simulink model "PV_PEM_direct_battery_passive"  (R2026a)
settings: Solver=VariableStepAuto  StopTime=sim_t
values from neighbouring files (symbols this model uses):
  Irr_stair_time = (0:Irr_stair_tsamp:sim_t)'    [PV_PEM_direct_battery_active.m]    (also in PV_PEM_direct_battery_passive.m = 0:Irr_stair_tsamp:sim_t; PV_PEM_indirect_battery.m; PV_PEM_reconfigurable_battery.m = (0 : Irr_stair_tsamp : sim_t)')
  Irr_stair_val = interp1(Irr_time, Irr_val, Irr_stair_time, 'linear', 0)    [PV_PEM_direct_battery_active.m]    (also in PV_PEM_direct_battery_passive.m; PV_PEM_indirect_battery.m; PV_PEM_reconfigurable_battery.m = interp1(Irr_time, Irr_val,  Irr_stair_time, 'linear', 0))
  Q_batt = 0.1    [PV_PEM_direct_battery_active.m]    (also in PV_PEM_direct_battery_passive.m; PV_PEM_indirect_battery.m; PV_PEM_reconfigurable_battery.m = 0.00694444444444)
  Ra_stack = Ra   * N    (= 0.02301)    [PV_PEM_direct_battery_active.m]    (also in PV_PEM_direct_battery_passive.m; PV_PEM_indirect_battery.m = 0.0177; PV_PEM_reconfigurable_battery.m = 0.02832)
  Rc_stack = Rc   * N    (= 0.0065)    [PV_PEM_direct_battery_active.m]    (also in PV_PEM_direct_battery_passive.m; PV_PEM_indirect_battery.m = 0.005; PV_PEM_reconfigurable_battery.m = 0.008)
  Rint_stack = Rint * N    (= 0.112749)    [PV_PEM_direct_battery_active.m]    (also in PV_PEM_direct_battery_passive.m; PV_PEM_indirect_battery.m = 0.08673; PV_PEM_reconfigurable_battery.m = 0.138768)
  sample_output_time = 1e-3    (= 0.001)    [PV_PEM_direct_battery_active.m]    (also in PV_PEM_direct_battery_passive.m = 0.0001; PV_PEM_indirect_battery.m = 0.01; PV_PEM_reconfigurable_battery.m = 0.00166666666667)
  SOC_max = 0.9    [PV_PEM_direct_battery_active.m]    (also in PV_PEM_direct_battery_passive.m = 90; PV_PEM_indirect_battery.m; PV_PEM_reconfigurable_battery.m = 90)
  SOC_min = 0.2    [PV_PEM_direct_battery_active.m]    (also in PV_PEM_direct_battery_passive.m = 20; PV_PEM_indirect_battery.m; PV_PEM_reconfigurable_battery.m = 20)
libraries: fl_lib x20, nesl_utility x15, simulink x3, ee_lib x3, batteryecm_lib x1
settings Model: Creator=hanna  LastModifiedBy=Diamantis
settings SimscapeCC: SimscapeNominalValues="[{\"value\":\"1\",\"unit\":\"A\"},{\"value\":\"1\",\"unit\":\"bar\"},{\"value\":\"1\",\"unit\":\"cm^2\"},{\"value\":\"1\",\"unit\":\"cm^3/s\"},{\"value\":\"1\",\"unit\":\"kJ/kg\"},{\"value\":\"1\",\"unit\":\"kW\"},{\"value\":\"1\",\"unit\":\"l\"},{\"value\":\"1\",\"unit\":\"N\"},{\"value\":\"1\",\"unit\":\"N*m\"},{\"value\":\"1\",\"unit\":\"V\"}]"  SimscapeLogType=none  SimscapeLogDataHistory=5000.0

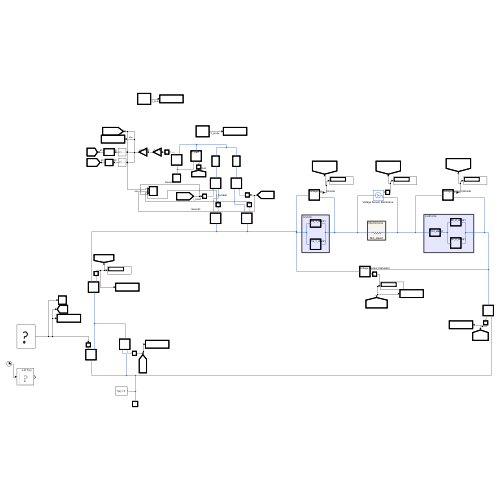
[thumbnail: Simulink's stored preview of the top-level diagram]
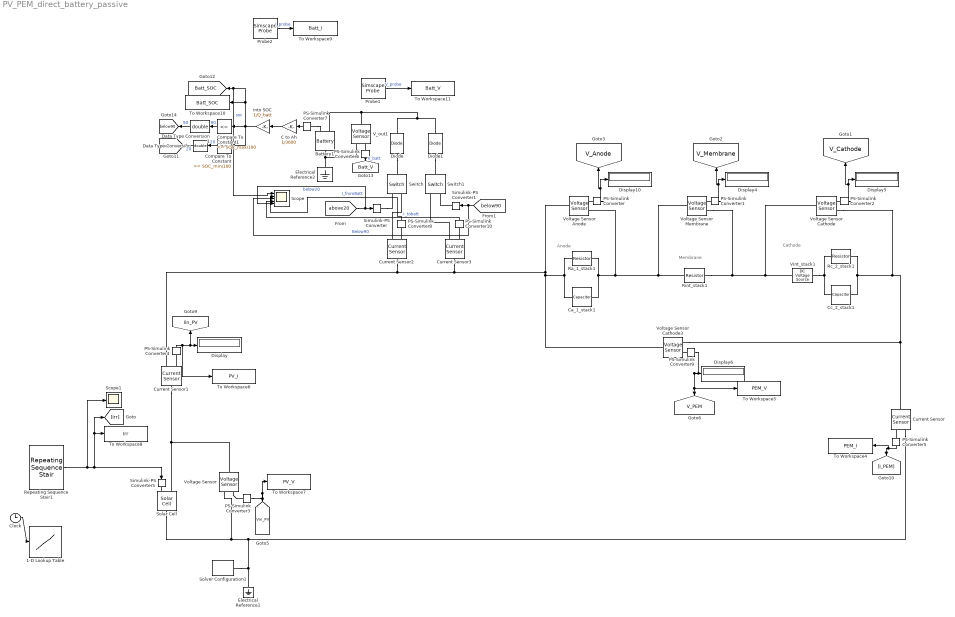
== system PV_PEM_direct_battery_passive ==
  note: Membrane
  note: Cathode
  note: Anode
  1-D Lookup Table : Lookup_n-D  NumberOfTableDimensions=1  BreakpointsForDimension1=Irr_stair_time  Table=Irr_stair_val  InternalRulePriority=Speed  RndMeth=Simplest
  Battery1 : batteryecm_lib/Battery  Vnom=V_batt_nom V  prm_dir=simscape.enum.battery.prm_dir.disabled  R1_dis=0.05 Ohm  R1_ch=0.05 Ohm  R1=0.01 Ohm  prm_AH=simscape.enum.battery.prm_AH.finite  AH=Q_batt A*hr  V1=11.5 V  AH1=Q_batt*(SOC_min/100) A*hr  prm_R2=simscape.enum.battery.prm_R2.disabled  R2=2000 Ohm  Tmeas=298.15 K  charge_measurement_port=simscape.enum.battery.enable.yes  prm_dyn=simscape.enum.battery.prm_dyn.off  Rp1=0.005 Ohm  tau1=30 s  Rp2=0.005 Ohm  tau2=30 s  Rp3=0.005 Ohm  tau3=30 s  Rp4=0.005 Ohm  tau4=30 s  Rp5=0.005 Ohm  tau5=30 s  prm_fade=simscape.enum.battery.prm_fade.disabled  N_fade=100  AH_fade=45 A*hr  R1_fade=2.02 Ohm  R1_ch_fade=2.02 Ohm  V1_fade=10.35 V  prm_age=simscape.enum.battery.prm_age.disabled  prm_age_OCV=simscape.enum.battery.prm_age_OCV.OCV  OCV_age=0.9  SOC_age=60  Tmeas_age=298.15 K  delta_time_age_vec=[0] d  temperature_age_vec=[273] K  OCV_scaling_age=2.2134e6  OCV_offset_age=1.632e6  temp_exp_age=0.515833569 V  t_exp_age=0.75  Vnom_T2=12 V  R1_T2=2.2 Ohm  R1_T2_dis=2.2 Ohm  R1_T2_ch=2.2 Ohm  V1_T2=11.4 V  R2_T2=2200 Ohm  Rp1_T2=0.005 Ohm  tau1_T2=30 s  Rp2_T2=0.005 Ohm  tau2_T2=30 s  Rp3_T2=0.005 Ohm  tau3_T2=30 s  Rp4_T2=0.005 Ohm  tau4_T2=30 s  Rp5_T2=0.005 Ohm  tau5_T2=30 s  Tmeas2=273.15 K  thermal_port=simscape.enum.thermaleffects.omit  thermal_mass=30000 J/K  i_specify=off  i_priority=None  i=0 A  i_nominal_specify=off  i_nominal_value=1  i_nominal_unit=A  v_specify=off  v_priority=None  v=0 V  v_nominal_specify=off  v_nominal_value=1  v_nominal_unit=V  charge_specify=on  charge_priority=High  charge=SOC_init A*hr  charge_nominal_specify=off  charge_nominal_value=1  charge_nominal_unit=A*hr  num_cycles_specify=off  num_cycles_priority=High  num_cycles=0  num_cycles_nominal_specify=off  num_cycles_nominal_value=1  num_cycles_nominal_unit=1  temperature_specify=off  temperature_priority=High  temperature=298.15 K  temperature_nominal_specify=off  temperature_nominal_value=1  temperature_nominal_unit=K
      settings: LibrarySourceBlock=batt_lib/Cells/Battery
  C to Ah : Gain  Gain=1/3600
  Ca_1_stack1 : fl_lib/Electrical/Electrical Elements/Capacitor  c=Ca_stack F  r=1e-6 Ohm  g=0 1/Ohm  i_specify=off  i_priority=None  i=0 A  i_nominal_specify=off  i_nominal_value=1  i_nominal_unit=A  v_specify=off  v_priority=None  v=0 V  v_nominal_specify=off  v_nominal_value=1  v_nominal_unit=V  vc_specify=off  vc_priority=High  vc=0 V  vc_nominal_specify=off  vc_nominal_value=1  vc_nominal_unit=V
  Cc_2_stack1 : fl_lib/Electrical/Electrical Elements/Capacitor  c=Cc_stack F  r=1e-6 Ohm  g=0 1/Ohm  i_specify=off  i_priority=None  i=0 A  i_nominal_specify=off  i_nominal_value=1  i_nominal_unit=A  v_specify=off  v_priority=None  v=0 V  v_nominal_specify=off  v_nominal_value=1  v_nominal_unit=V  vc_specify=off  vc_priority=High  vc=0 V  vc_nominal_specify=off  vc_nominal_value=1  vc_nominal_unit=V
  Clock : Clock
  Compare To Constant : simulink/Logic and Bit Operations/Compare To Constant  relop=>=  const=SOC_min/100  OutDataTypeStr=boolean
  Compare To Constant1 : simulink/Logic and Bit Operations/Compare To Constant  relop=<=  const=SOC_max/100  OutDataTypeStr=boolean
  Current Sensor{,1..3} (4 alike) : fl_lib/Electrical/Electrical Sensors/Current Sensor
  Data Type Conversion : DataTypeConversion  OutDataTypeStr=double  SaturateOnIntegerOverflow=off  RndMeth=Floor
  Data Type Conversion1 : DataTypeConversion  OutDataTypeStr=double  SaturateOnIntegerOverflow=off  RndMeth=Floor
  Diode : ee_lib/Semiconductors & Converters/Diode  ModelType=ee.enum.diode.modelType.pwl  TableType=ee.enum.diode.tableType.IfMat  IfMat=[.07, .12, .19, 1.75, 4.24, 7.32, 11.2; .16, .3, .72, 2.14, 5.02, 8.35, 13.12] A  VfMat=[.9, 1.15, 1.25, 1.5, 1.75, 2.17, 2.6, 2.85; .58, .68, .75, 1.1, 1.38, 1.77, 2.27, 2.7] V  TjVec=[25, 125] degC  VfVec=[.5, .7, .9, 1.3, 1.7, 2.1, 2.5] V  IfVec=[.1, .2, .5, 1, 2, 4, 7, 10] A  IrMat=[1e-06, 2e-06, 5e-06, 1e-05, 2.5e-05, 5e-05, .0001; 2e-06, 5e-06, 1e-05, 4e-05, 8e-05, .0002, .0005] A  VrMat=[10, 100, 200, 250, 300, 325, 350; 10, 70, 160, 220, 270, 300, 320] V  VrVec=[10, 20, 40, 50, 70, 80, 100] V  IrVec=[1e-06, 2e-06, 5e-06, 1e-05, 2e-05, 5e-05, .0001] A  Vf=0.6 V  Ron=0.3 Ohm  Goff=1e-8 S  prmExp=ee.enum.diode.expParam.useTwo  I12=[.0137, .545] A  V12=[.6, .7] V  RS=0 Ohm  Tmeas=298.15 K  IS=1e-12 A  ec=1  I1=0.0137 A  V1=0.6 V  N_series=1  N_parallel=1  ZenerEnable=false  Rz=0.3 Ohm  BV=inf V  C_param=ee.enum.diode.capParam.fixed  CJ=0 pF  CJ0=5 pF  Vvec=[.1, 10, 100] V  Cvec=[3.5, 1, .4] pF  VJ=1 V  Mgrad=0.5  FC=0.5  Q_param=ee.enum.diode.recoveryParam.off  iRM=-7.15 A  iF=4 A  didt=-750 A/us  trr_factor=3  trr=115 ns  Qrr=150 nA*s  Vr=-600 V  Ls=150 nH  Erec=0.03 J  TT=50 ns  tau=100 ns  T_param=ee.enum.diode.temperatureParam.off  Tdevice=298.15 K  I1_T2=0.245 A  V1_T2=0.5 V  IS_T2=1.25e-7 A  Tmeas2=125 degC  XTI_param=ee.enum.diode.xtiParam.pn  XTI=3  EG_param=ee.enum.diode.egapParam.material_si  EG=1.11 eV  dBVdT=0 V/K  enable_fault_input=simscape.enum.onoff.off  i_specify=off  i_priority=None  i=0 A  i_nominal_specify=off  i_nominal_value=1  i_nominal_unit=A  v_specify=off  v_priority=None  v=0 V  v_nominal_specify=off  v_nominal_value=1  v_nominal_unit=V  v_capacitor_specify=off  v_capacitor_priority=None  v_capacitor=0 V  v_capacitor_nominal_specify=off  v_capacitor_nominal_value=1  v_capacitor_nominal_unit=V  Qj_specify=off  Qj_priority=High  Qj=0 C  Qj_nominal_specify=off  Qj_nominal_value=1  Qj_nominal_unit=C  i_diode_specify=off  i_diode_priority=None  i_diode=0 A  i_diode_nominal_specify=off  i_diode_nominal_value=1  i_diode_nominal_unit=A  v_diode_specify=off  v_diode_priority=None  v_diode=0 V  v_diode_nominal_specify=off  v_diode_nominal_value=1  v_diode_nominal_unit=V  i_capacitor_specify=off  i_capacitor_priority=None  i_capacitor=0 A  i_capacitor_nominal_specify=off  i_capacitor_nominal_value=1  i_capacitor_nominal_unit=A  fidelity_level=ee.enum.diode.fidelity.includeChargeDyn  rec_loss_model=ee.enum.diode.reverseRecoveryModel.fixed  ErecVal=0 J  scaleWithIandV=true  ErecMat=zeros(2, 3) J  ErecMat3D=zeros(2, 3, 2) J  TjrecVec=[298.15, 398.15] K  IfrecVec=[.1, 1, 10] A  IrecVal=10 A  VrecVal=10 V  VrecVec=[0, 100] V  tFilter=1 / 1000 / 100 s  thermal_network_parameterization=ee.enum.thermalNetworkTopology.junctionCase  Rth=[0, 10] K/W  Rth_Cauer=[1, 3, 10] K/W  Rth_Foster=[.08, .14, .22, .16] K/W  thermal_mass_parameterization=ee.enum.thermalNetwork.timeconstant  thermal_mass=[0, 1] J/K  thermal_mass_Cauer=[.1, .3, 1] J/K  thermal_mass_Foster=[.001, .005, .05, .5] J/K  thermal_time_constant=[0, 10] s  thermal_time_constant_Cauer=[1, 3, 10] s  thermal_time_constant_Foster=[7e-05, .0007, .01, .08] s  thermal_mass_initial_temperatures=[25, 25] degC  thermal_mass_initial_temperatures_Cauer=[25, 25, 25] degC  junction_thermal_mass=0.01 J/K  Tvec_initial_Foster=[25, 25, 25, 25] degC  no_thermal_network=0  junction_temperature_specify=off  junction_temperature_priority=None  junction_temperature=25 degC  junction_temperature_nominal_specify=off  junction_temperature_nominal_value=1  junction_temperature_nominal_unit=degC
  Diode1 : ee_lib/Semiconductors & Converters/Diode  ModelType=ee.enum.diode.modelType.pwl  TableType=ee.enum.diode.tableType.IfMat  IfMat=[.07, .12, .19, 1.75, 4.24, 7.32, 11.2; .16, .3, .72, 2.14, 5.02, 8.35, 13.12] A  VfMat=[.9, 1.15, 1.25, 1.5, 1.75, 2.17, 2.6, 2.85; .58, .68, .75, 1.1, 1.38, 1.77, 2.27, 2.7] V  TjVec=[25, 125] degC  VfVec=[.5, .7, .9, 1.3, 1.7, 2.1, 2.5] V  IfVec=[.1, .2, .5, 1, 2, 4, 7, 10] A  IrMat=[1e-06, 2e-06, 5e-06, 1e-05, 2.5e-05, 5e-05, .0001; 2e-06, 5e-06, 1e-05, 4e-05, 8e-05, .0002, .0005] A  VrMat=[10, 100, 200, 250, 300, 325, 350; 10, 70, 160, 220, 270, 300, 320] V  VrVec=[10, 20, 40, 50, 70, 80, 100] V  IrVec=[1e-06, 2e-06, 5e-06, 1e-05, 2e-05, 5e-05, .0001] A  Vf=0.6 V  Ron=0.3 Ohm  Goff=1e-8 S  prmExp=ee.enum.diode.expParam.useTwo  I12=[.0137, .545] A  V12=[.6, .7] V  RS=0 Ohm  Tmeas=298.15 K  IS=1e-12 A  ec=1  I1=0.0137 A  V1=0.6 V  N_series=1  N_parallel=1  ZenerEnable=false  Rz=0.3 Ohm  BV=inf V  C_param=ee.enum.diode.capParam.fixed  CJ=0 pF  CJ0=5 pF  Vvec=[.1, 10, 100] V  Cvec=[3.5, 1, .4] pF  VJ=1 V  Mgrad=0.5  FC=0.5  Q_param=ee.enum.diode.recoveryParam.off  iRM=-7.15 A  iF=4 A  didt=-750 A/us  trr_factor=3  trr=115 ns  Qrr=150 nA*s  Vr=-600 V  Ls=150 nH  Erec=0.03 J  TT=50 ns  tau=100 ns  T_param=ee.enum.diode.temperatureParam.off  Tdevice=298.15 K  I1_T2=0.245 A  V1_T2=0.5 V  IS_T2=1.25e-7 A  Tmeas2=125 degC  XTI_param=ee.enum.diode.xtiParam.pn  XTI=3  EG_param=ee.enum.diode.egapParam.material_si  EG=1.11 eV  dBVdT=0 V/K  enable_fault_input=simscape.enum.onoff.off  i_specify=off  i_priority=None  i=0 A  i_nominal_specify=off  i_nominal_value=1  i_nominal_unit=A  v_specify=off  v_priority=None  v=0 V  v_nominal_specify=off  v_nominal_value=1  v_nominal_unit=V  v_capacitor_specify=off  v_capacitor_priority=None  v_capacitor=0 V  v_capacitor_nominal_specify=off  v_capacitor_nominal_value=1  v_capacitor_nominal_unit=V  Qj_specify=off  Qj_priority=High  Qj=0 C  Qj_nominal_specify=off  Qj_nominal_value=1  Qj_nominal_unit=C  i_diode_specify=off  i_diode_priority=None  i_diode=0 A  i_diode_nominal_specify=off  i_diode_nominal_value=1  i_diode_nominal_unit=A  v_diode_specify=off  v_diode_priority=None  v_diode=0 V  v_diode_nominal_specify=off  v_diode_nominal_value=1  v_diode_nominal_unit=V  i_capacitor_specify=off  i_capacitor_priority=None  i_capacitor=0 A  i_capacitor_nominal_specify=off  i_capacitor_nominal_value=1  i_capacitor_nominal_unit=A  fidelity_level=ee.enum.diode.fidelity.includeChargeDyn  rec_loss_model=ee.enum.diode.reverseRecoveryModel.fixed  ErecVal=0 J  scaleWithIandV=true  ErecMat=zeros(2, 3) J  ErecMat3D=zeros(2, 3, 2) J  TjrecVec=[298.15, 398.15] K  IfrecVec=[.1, 1, 10] A  IrecVal=10 A  VrecVal=10 V  VrecVec=[0, 100] V  tFilter=1 / 1000 / 100 s  thermal_network_parameterization=ee.enum.thermalNetworkTopology.junctionCase  Rth=[0, 10] K/W  Rth_Cauer=[1, 3, 10] K/W  Rth_Foster=[.08, .14, .22, .16] K/W  thermal_mass_parameterization=ee.enum.thermalNetwork.timeconstant  thermal_mass=[0, 1] J/K  thermal_mass_Cauer=[.1, .3, 1] J/K  thermal_mass_Foster=[.001, .005, .05, .5] J/K  thermal_time_constant=[0, 10] s  thermal_time_constant_Cauer=[1, 3, 10] s  thermal_time_constant_Foster=[7e-05, .0007, .01, .08] s  thermal_mass_initial_temperatures=[25, 25] degC  thermal_mass_initial_temperatures_Cauer=[25, 25, 25] degC  junction_thermal_mass=0.01 J/K  Tvec_initial_Foster=[25, 25, 25, 25] degC  no_thermal_network=0  junction_temperature_specify=off  junction_temperature_priority=None  junction_temperature=25 degC  junction_temperature_nominal_specify=off  junction_temperature_nominal_value=1  junction_temperature_nominal_unit=degC
  Display{,4..6,10} (5 alike) : Display
  Electrical Reference2 : fl_lib/Electrical/Electrical Elements/Electrical Reference
  Electrical Reference1 : fl_lib/Electrical/Electrical Elements/Electrical Reference
  PS-Simulink Converter{,1..2,5..7,9} (7 alike) : nesl_utility/PS-Simulink Converter  PhysicalDomain=network_engine_domain  SubClassName=ps_output  LeftPortType=input  RightPortType=output  PseudoPeriodic=off  Frequencies=[]  VectorFormat=inherit  Unit=inherit  AffineConversion=off
  PS-Simulink Converter10 : nesl_utility/PS-Simulink Converter  PhysicalDomain=network_engine_domain  SubClassName=ps_output  LeftPortType=input  RightPortType=output  PseudoPeriodic=off  Frequencies=[]  VectorFormat=1-D array  Unit=A  AffineConversion=off
  PS-Simulink Converter3 : nesl_utility/PS-Simulink Converter  PhysicalDomain=network_engine_domain  SubClassName=ps_output  LeftPortType=input  RightPortType=output  PseudoPeriodic=off  Frequencies=[]  VectorFormat=1-D array  Unit=V  AffineConversion=off
  PS-Simulink Converter4 : nesl_utility/PS-Simulink Converter  PhysicalDomain=network_engine_domain  SubClassName=ps_output  LeftPortType=input  RightPortType=output  PseudoPeriodic=off  Frequencies=[]  VectorFormat=1-D array  Unit=A  AffineConversion=off
  PS-Simulink Converter8 : nesl_utility/PS-Simulink Converter  PhysicalDomain=network_engine_domain  SubClassName=ps_output  LeftPortType=input  RightPortType=output  PseudoPeriodic=off  Frequencies=[]  VectorFormat=1-D array  Unit=A  AffineConversion=off
  Probe1 : SimscapeProbe  BoundBlock=499  Variables="{\"i\":{\"Probing\":\"OFF\"},\"n.v\":{\"Probing\":\"OFF\"},\"p.v\":{\"Probing\":\"OFF\"},\"v\":{\"Probing\":\"ON\"}}"
  Probe2 : SimscapeProbe  BoundBlock=499  Variables="{\"i\":{\"Probing\":\"ON\"}}"
  Ra_1_stack1 : fl_lib/Electrical/Electrical Elements/Resistor  R=Ra_stack Ohm  i_specify=off  i_priority=None  i=0 A  i_nominal_specify=off  i_nominal_value=1  i_nominal_unit=A  v_specify=off  v_priority=None  v=0 V  v_nominal_specify=off  v_nominal_value=1  v_nominal_unit=V
  Rc_2_stack1 : fl_lib/Electrical/Electrical Elements/Resistor  R=Rc_stack Ohm  i_specify=off  i_priority=None  i=0 A  i_nominal_specify=off  i_nominal_value=1  i_nominal_unit=A  v_specify=off  v_priority=None  v=0 V  v_nominal_specify=off  v_nominal_value=1  v_nominal_unit=V
  Repeating Sequence Stair1 : simulink/Sources/Repeating Sequence Stair  OutValues=Irr_stair_val  tsamp=Irr_stair_tsamp  OutMin=[]  OutMax=[]  OutDataTypeStr=double  OutputDataTypeScalingMode=double  OutDataType=fixdt(0,8)  ConRadixGroup=Best Precision: Vector-wise  OutScaling=2^-12
  Rint_stack1 : fl_lib/Electrical/Electrical Elements/Resistor  R=Rint_stack Ohm  i_specify=off  i_priority=None  i=0 A  i_nominal_specify=off  i_nominal_value=1  i_nominal_unit=A  v_specify=off  v_priority=None  v=0 V  v_nominal_specify=off  v_nominal_value=1  v_nominal_unit=V
  Scope : Scope  NumInputPorts=5
      settings: ActiveDisplayYMinimum=0.599999044089406  ActiveDisplayYMaximum=0.60000010621228816  DataLoggingVariableName=ScopeData4
  Scope1 : Scope
      settings: ActiveDisplayYMinimum=-124.99999999999997  ActiveDisplayYMaximum=1125
  Simulink-PS Converter : nesl_utility/Simulink-PS Converter  PhysicalDomain=network_engine_domain  SubClassName=ps_input  LeftPortType=input  RightPortType=output  PseudoPeriodic=off  Frequencies=[]  NoiseDistribution=none  NoiseParameters=[]  Unit=1  AffineConversion=off  FilteringAndDerivatives=provide  SimscapeFilterOrder=1  InputFilterTimeConstant=0.001  UdotUserProvided=0
  Simulink-PS Converter1 : nesl_utility/Simulink-PS Converter  PhysicalDomain=network_engine_domain  SubClassName=ps_input  LeftPortType=input  RightPortType=output  PseudoPeriodic=off  Frequencies=[]  NoiseDistribution=none  NoiseParameters=[]  Unit=1  AffineConversion=off  FilteringAndDerivatives=provide  SimscapeFilterOrder=1  InputFilterTimeConstant=0.001  UdotUserProvided=0
  Simulink-PS Converter5 : nesl_utility/Simulink-PS Converter  PhysicalDomain=network_engine_domain  SubClassName=ps_input  LeftPortType=input  RightPortType=output  PseudoPeriodic=off  Frequencies=[]  NoiseDistribution=none  NoiseParameters=[]  Unit=1  AffineConversion=off  FilteringAndDerivatives=provide  SimscapeFilterOrder=1  InputFilterTimeConstant=0.001  UdotUserProvided=0
  Solar Cell : ee_lib/Sources/Solar Cell  PartSpecification="{\"CollectionId\":\"SimscapeElectrical\",\"CollectionVersion\":\"1.0.0\",\"DatasetId\":\"Amerisolar|AS_6M30_HC_320W|simscape.electrical.solarCell\",\"DisplayName\":\"Amerisolar:AS_6M30_HC_320W\"}"  prm=3  Isc=10.14 % Datasheet derived A  Voc=0.67 % Datasheet derived V  Is=3.24823447983853e-07 % Datasheet derived A  Is2=9.37081970792037e-10 % Datasheet derived A  Iph=10.140005507508 % Datasheet derived A  Ir0=1000 % Datasheet derived W/m^2  ec=1.51118472243322 % Datasheet derived  N2=2.60259908345858 % Datasheet derived  Rs=1.94548269975201e-05 % Datasheet derived Ohm  Rp=682.95993142779 % Datasheet derived Ohm  N_series=Ns_cell % Datasheet derived  N_parallel=Np_cell % Datasheet derived  TIPH1=0.000499942933005141 % Datasheet derived 1/K  EG=1.12 % Datasheet derived eV  TXIS1=4.23641510120988 % Datasheet derived  TXIS2=16.2689137700667 % Datasheet derived  TRS1=0.243341028305912 % Datasheet derived  TRP1=0 % Parameter not set  Tmeas=25 % Datasheet derived degC  TFIXED=25 % Datasheet derived degC  thermal_mass=100 % Parameter not set J/K  initial_temperature=25 degC
      settings: AttributesFormatString=Amerisolar:AS_6M30_HC_320W
  Solver Configuration1 : nesl_utility/Solver Configuration  PhysicalDomain=network_engine_domain  SubClassName=solver  LeftPortType=input  RightPortType=generic  Tones=[]  Harmonics=[]  SimulateNoise=off  Profile=off  UseLocalSampling=off  EnableSwitchedLinearOptims=on  FrequencyDomain=off  UseCCode=off  RelTol=0.001  AbsTol=0.001  MinStep=1e-09  ToWorkspace=off  RevertToSquareIcSolve=off  NumHomotopyIterations=100  PhasorMode=off  PhasorModeNumHarmonics=1  ConsistencySolver=NEWTON_XTOL_AFTER_FTOL  CanonicalOrdering=UNORDERED  OptimizeIntermediates=UNOPTIMIZED  IndexReductionMethod=DerivativeReplacement  DoDC=off  ResidualTolerance=1e-09  ConsistencyTolSource=GLOBAL  ConsistencyAbsTol=0.001  ConsistencyRelTol=0.001  ConsistencyTolFactor=0.001  UseLocalSolver=off  LocalSolverChoice=NE_BACKWARD_EULER_ADVANCER  ResolveIndetEquations=on  FunctionEvalNumThread=1  LocalSolverSampleTime=0.001  DoFixedCost=off  MaxNonlinIter=3  MaxModeIter=2  ComputeImpulses=off  ImpulseIterations=2  LinearAlgebra=auto  LinearAlgebraNumThread=0  EquationFormulation=NE_TIME_EF  DelaysMemoryBudget=1024  AutomaticFiltering=on  FilteringTimeConstant=0.001  PartitionStorageMethod=AS_NEEDED  PartitionMemoryBudget=1024  PartitionMethod=ROBUST  MultibodyUseLocalSolver=off  MultibodyLocalSolverChoice=ODE1  MultibodyLocalSolverSampleTime=0.001
  Switch : fl_lib/Electrical/Electrical Elements/Switch  R_closed=0.01 Ohm  G_open=1e-8 1/Ohm  Threshold=0.5  i_specify=off  i_priority=None  i=0 A  i_nominal_specify=off  i_nominal_value=1  i_nominal_unit=A  v_specify=off  v_priority=None  v=0 V  v_nominal_specify=off  v_nominal_value=1  v_nominal_unit=V
  Switch1 : fl_lib/Electrical/Electrical Elements/Switch  R_closed=0.01 Ohm  G_open=1e-8 1/Ohm  Threshold=0.5  i_specify=off  i_priority=None  i=0 A  i_nominal_specify=off  i_nominal_value=1  i_nominal_unit=A  v_specify=off  v_priority=None  v=0 V  v_nominal_specify=off  v_nominal_value=1  v_nominal_unit=V
  To Workspace10 : ToWorkspace  VariableName=Batt_SOC  SaveFormat=Timeseries  SampleTime=sample_output_time
  To Workspace11 : ToWorkspace  VariableName=Batt_V  SaveFormat=Timeseries  SampleTime=sample_output_time
  To Workspace4 : ToWorkspace  VariableName=PEM_I  SaveFormat=Timeseries  SampleTime=sample_output_time
  To Workspace5 : ToWorkspace  VariableName=PEM_V  SaveFormat=Timeseries  SampleTime=sample_output_time
  To Workspace6 : ToWorkspace  VariableName=PV_I  SaveFormat=Timeseries  SampleTime=sample_output_time
  To Workspace7 : ToWorkspace  VariableName=PV_V  SaveFormat=Timeseries  SampleTime=sample_output_time
  To Workspace8 : ToWorkspace  VariableName=Irr  SaveFormat=Timeseries  SampleTime=sample_output_time
  To Workspace9 : ToWorkspace  VariableName=Batt_I  SaveFormat=Timeseries  SampleTime=sample_output_time
  V_out1 : fl_lib/Electrical/Electrical Sensors/Voltage Sensor
  Vint_stack1 : fl_lib/Electrical/Electrical Sources/DC Voltage Source  v0=Vint_stack V
  Voltage Sensor : fl_lib/Electrical/Electrical Sensors/Voltage Sensor
  Voltage Sensor Anode : fl_lib/Electrical/Electrical Sensors/Voltage Sensor
  Voltage Sensor Cathode : fl_lib/Electrical/Electrical Sensors/Voltage Sensor
  Voltage Sensor Cathode3 : fl_lib/Electrical/Electrical Sensors/Voltage Sensor
  Voltage Sensor Membrane : fl_lib/Electrical/Electrical Sensors/Voltage Sensor
  into SOC : Gain  Gain=1/Q_batt
  tag scope: Batt_SOC=global, Batt_V=global, Iin_PV=global, V_Anode=global, V_Cathode=global, V_Membrane=global, V_PEM=global, Vin_PV=global, above20=global, below90=global
  wires:
  Repeating Sequence Stair1/1 -> Simulink-PS Converter5/1, To Workspace8/1, [Irr], Scope1/1
  Clock/1 -> 1-D Lookup Table/1
  PS-Simulink Converter1/1 -> [V_Membrane], Display4/1
  PS-Simulink Converter9/1 -> To Workspace5/1, [V_PEM], Display6/1
  PS-Simulink Converter/1 -> [V_Anode], Display10/1
  PS-Simulink Converter2/1 -> [V_Cathode], Display5/1
  PS-Simulink Converter4/1 -> To Workspace6/1, [Iin_PV], Display/1
  PS-Simulink Converter5/1 -> To Workspace4/1, [I_PEM]
  PS-Simulink Converter3/1 -> To Workspace7/1, [Vin_PV]
  Compare To Constant1/1 -> Data Type Conversion1/1  "90"
  Compare To Constant/1 -> Data Type Conversion/1  "20"
  into SOC/1 -> Compare To Constant1/1, To Workspace10/1, Scope/1, [Batt_SOC], Compare To Constant/1  "soc"
  Data Type Conversion1/1 -> [below90]  "90"
  C to Ah/1 -> into SOC/1
  Probe1/1 -> To Workspace11/1  "V_probe"
  PS-Simulink Converter7/1 -> C to Ah/1
  PS-Simulink Converter6/1 -> [Batt_V]  "V_batt"
  Data Type Conversion/1 -> [above20]  "20"
  Probe2/1 -> To Workspace9/1  "I_probe"
  [above20] -> Scope/5, Simulink-PS Converter/1  "below20"
  [below90] -> Scope/3, Simulink-PS Converter1/1  "Below90"
  PS-Simulink Converter10/1 -> Scope/4  "I_tobatt"
  PS-Simulink Converter8/1 -> Scope/2  "I_fromBatt"
  connections:
  Solver Configuration1/RConn1 -- Voltage Sensor/RConn2 -- Solar Cell/RConn1 -- Current Sensor/RConn2 -- Electrical Reference1/LConn1
  Simulink-PS Converter5/RConn1 -- Solar Cell/LConn1
  Current Sensor1/LConn1 -- Voltage Sensor/LConn1 -- Solar Cell/LConn2
  Voltage Sensor Anode/RConn2 -- Ra_1_stack1/RConn1 -- Ca_1_stack1/RConn1 -- Rint_stack1/LConn1 -- Voltage Sensor Membrane/LConn1
  Voltage Sensor Membrane/RConn2 -- Voltage Sensor Cathode/LConn1 -- Vint_stack1/LConn1 -- Rint_stack1/RConn1
  Cc_2_stack1/RConn1 -- Rc_2_stack1/RConn1 -- Current Sensor/LConn1 -- Voltage Sensor Cathode3/RConn2 -- Voltage Sensor Cathode/RConn2
  Cc_2_stack1/LConn1 -- Vint_stack1/RConn1 -- Rc_2_stack1/LConn1
  Voltage Sensor Cathode3/RConn1 -- PS-Simulink Converter9/LConn1
  Voltage Sensor Membrane/RConn1 -- PS-Simulink Converter1/LConn1
  Voltage Sensor Cathode/RConn1 -- PS-Simulink Converter2/LConn1
  Voltage Sensor Anode/RConn1 -- PS-Simulink Converter/LConn1
  Current Sensor1/RConn1 -- PS-Simulink Converter4/LConn1
  PS-Simulink Converter5/LConn1 -- Current Sensor/RConn1
  PS-Simulink Converter3/LConn1 -- Voltage Sensor/RConn1
  V_out1/LConn1 -- Diode/LConn1 -- Diode1/RConn1 -- Battery1/LConn1
  Battery1/RConn1 -- V_out1/RConn2 -- Electrical Reference2/LConn1
  V_out1/RConn1 -- PS-Simulink Converter6/LConn1
  PS-Simulink Converter7/LConn1 -- Battery1/LConn2
  Diode/RConn1 -- Switch/LConn1
  Diode1/LConn1 -- Switch1/LConn1
  Voltage Sensor Cathode3/LConn1 -- Current Sensor1/RConn2 -- Current Sensor2/LConn1 -- Current Sensor3/LConn1 -- Voltage Sensor Anode/LConn1 -- Ca_1_stack1/LConn1 -- Ra_1_stack1/LConn1
  Simulink-PS Converter/RConn1 -- Switch/RConn1
  Simulink-PS Converter1/RConn1 -- Switch1/RConn1
  Current Sensor2/RConn1 -- PS-Simulink Converter8/LConn1
  Current Sensor3/RConn1 -- PS-Simulink Converter10/LConn1
  Current Sensor2/RConn2 -- Switch/RConn2
  Current Sensor3/RConn2 -- Switch1/RConn2
